simulink model "neuron_intandfire"  (Simulink 6.3)
settings: Solver=ode45  StartTime=0.0  StopTime=40  FixedStep=0.01  MaxStep=0.001  RelTol=1e-3
PreLoadFcn:
  | a=[-0.1 0.1];
libraries: simulink x1
settings Model: LastModifiedBy=sglasauer
settings DataIOCC: LimitDataPoints=off

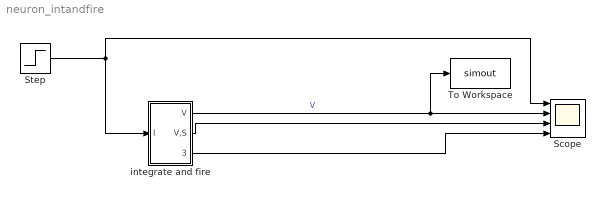
== system neuron_intandfire ==
  Scope : Scope  NumInputPorts=4
      settings: YMin=0~-59~-60~0  YMax=20~-49~50~100
  Step : Step  After=20  SampleTime=0
  To Workspace : ToWorkspace  VariableName=simout  SampleTime=-1  SaveFormat=Array
  integrate and fire : Subsystem  mask{th=-50+a}
      mask prompts: th "Threshold"
      mask Display: disp('I & F')
  wires:
  Step/1 -> Scope/1, integrate and fire/1(I)
  integrate and fire/2(V,S) -> Scope/3
  integrate and fire/1(V) -> Scope/2, To Workspace/1  "V"
  integrate and fire/3(Spikes) -> Scope/4

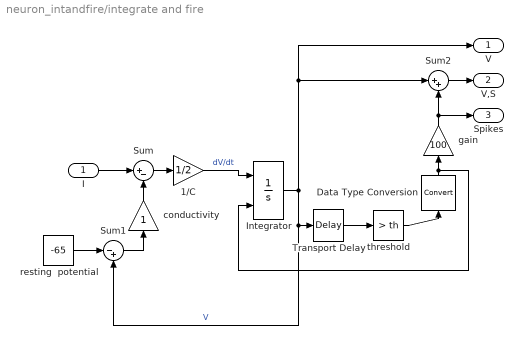
== system neuron_intandfire/integrate and fire ==
  I : Inport
  1/C : Gain  Gain=1/2
  Data Type Conversion : DataTypeConversion  Orientation=up  OutDataTypeMode=double
  Integrator : Integrator  ExternalReset=rising  InitialCondition=-55
  Sum : Sum  Inputs=|+-
  Sum1 : Sum  Inputs=|-+
  Sum2 : Sum  Inputs=|++
  Transport Delay : TransportDelay  DelayTime=0.1  InitialOutput=-65
  conductivity : Gain  Orientation=up
  gain : Gain  Orientation=up  Gain=100
  resting  potential : Constant  Value=-65
  threshold : simulink/Logic and Bit Operations/Compare To Constant  relop=>  const=th  LogicOutDataTypeMode=boolean
  V : Outport
  V,S : Outport  Port=2
  Spikes : Outport  Port=3
  wires:
  Sum1/1 -> conductivity/1
  conductivity/1 -> Sum/2
  resting  potential/1 -> Sum1/1
  Sum/1 -> 1/C/1
  1/C/1 -> Integrator/1  "dV/dt"
  Integrator/1 -> Transport Delay/1, Sum1/2, Sum2/1, V/1  "V"
  threshold/1 -> Data Type Conversion/1
  Transport Delay/1 -> threshold/1
  gain/1 -> Sum2/2, Spikes/1
  Data Type Conversion/1 -> gain/1, Integrator/2
  I/1 -> Sum/1
  Sum2/1 -> V,S/1
